simulink model "corBO"  (R2016b)
settings: Solver=VariableStepAuto  StartTime=0.0  StopTime=10.0  RelTol=1e-3
values from neighbouring files (symbols this model uses):
  f = 1    [Cons.m]
  Ki = 42.4/1000    (= 0.0424)    [Cons.m]
  Kred = 35.9    [Cons.m]
  meq = 120    [Cons.m]
  rpignon = 21*0.8/(2*1000)    (= 0.0084)    [Cons.m]
settings Model: Creator=canar  LastModifiedBy=canar

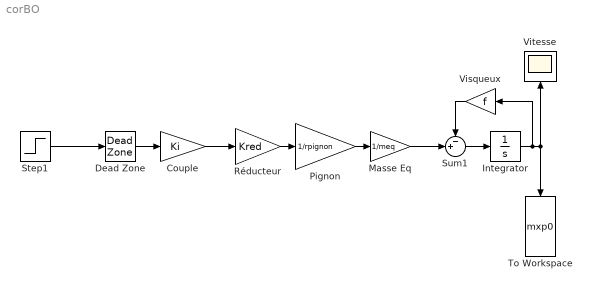
== system corBO ==
  Couple : Gain  Gain=Ki
  Dead Zone : DeadZone  LowerValue=-0.05  UpperValue=0.05  SaturateOnIntegerOverflow=on
  Integrator : Integrator
  Masse Eq : Gain  Gain=1/meq
  Pignon : Gain  Gain=1/rpignon
  Réducteur : Gain  Gain=Kred
  Step1 : Step  Time=0.1  After=0.2  SampleTime=0
  Sum1 : Sum  Inputs=-+|
  To Workspace : ToWorkspace  VariableName=mxp0  SaveFormat=Timeseries  SampleTime=-1
  Visqueux : Gain  Gain=f
  Vitesse : Scope
  wires:
  Pignon/1 -> Masse Eq/1
  Integrator/1 -> Visqueux/1, To Workspace/1, Vitesse/1
  Sum1/1 -> Integrator/1
  Visqueux/1 -> Sum1/1
  Masse Eq/1 -> Sum1/2
  Réducteur/1 -> Pignon/1
  Step1/1 -> Dead Zone/1
  Couple/1 -> Réducteur/1
  Dead Zone/1 -> Couple/1
